simulink model "Tf_model"  (R2024a)
settings: Solver=VariableStepAuto  StartTime=0.0  StopTime=10.0  RelTol=1e-3
undefined symbols (not defined in the file): b, F, k, M
settings Model: Creator=alisr_qxy0y9  LastModifiedBy=alisr_qxy0y9

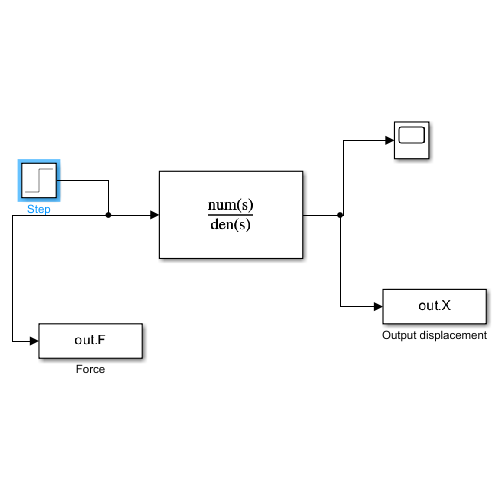
[thumbnail: Simulink's stored preview of the top-level diagram]
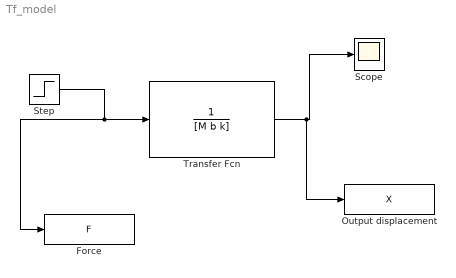
== system Tf_model ==
  Force : ToWorkspace  VariableName=F  SaveFormat=Timeseries  SampleTime=-1
  Output displacement : ToWorkspace  VariableName=X  SaveFormat=Timeseries  SampleTime=-1
  Scope : Scope
  Step : Step  Time=F  SampleTime=0
  Transfer Fcn : TransferFcn  Denominator=[M b k]
  wires:
  Step/1 -> Transfer Fcn/1, Force/1
  Transfer Fcn/1 -> Output displacement/1, Scope/1
